simulink model "Madgwick"  (R2018a)
settings: Solver=FixedStepAuto  StartTime=0.0  StopTime=10.0  RelTol=1e-3
PreLoadFcn:
  | modelDir = fileparts(get_param(bdroot, 'FileName'));
  | addpath(fullfile(modelDir,'../../Parameters'));
  | addpath(fullfile(modelDir,'../../Estimators/Madgwick'));
  | 
  | Parameters_Estimators
  | Parameters_Simulation
InitFcn:
  | Parameters_Estimators
  | Parameters_Simulation
undefined symbols (not defined in the file or in its folder): est_q_init, Ts
settings Model: Creator=Thomas  LastModifiedBy=Thomas

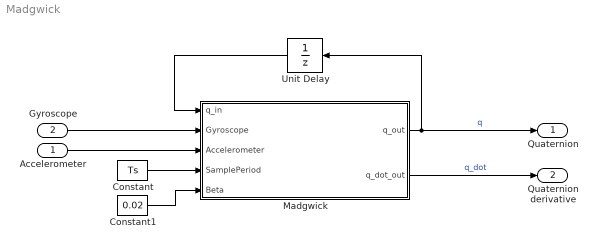
== system Madgwick ==
  Accelerometer : Inport
  Gyroscope : Inport  Port=2
  Constant : Constant  Value=Ts
  Constant1 : Constant  Value=0.02
  Madgwick : MATLAB Function  TreatAsAtomicUnit=on
  Unit Delay : UnitDelay  InitialCondition=est_q_init  SampleTime=Ts
  Quaternion : Outport
  Quaternion derivative : Outport  Port=2
  wires:
  Gyroscope/1 -> Madgwick/2(Gyroscope)
  Constant/1 -> Madgwick/4(SamplePeriod)
  Unit Delay/1 -> Madgwick/1(q_in)
  Accelerometer/1 -> Madgwick/3(Accelerometer)
  Madgwick/1(q_out) -> Unit Delay/1, Quaternion/1  "q"
  Madgwick/2(q_dot_out) -> Quaternion derivative/1  "q_dot"
  Constant1/1 -> Madgwick/5(Beta)

== matlab function Madgwick/Madgwick ==
  data: q_in input size=4; q_out output size=4; Gyroscope input size=3; Accelerometer input size=3; q_dot_out output size=4; SamplePeriod input; Beta input
function [q_out, q_dot_out] = MadgwickAHRS(q_in, Gyroscope, Accelerometer, SamplePeriod, Beta)           
    
    q = q_in';    

    % Normalise accelerometer measurement
    if(norm(Accelerometer) == 0)
        disp('ERROR - NaN in Madgwick');
        q_out = q';
        q_dot_out = [0,0,0,0]';
        return;
    end	% handle NaN
    Accelerometer = Accelerometer / norm(Accelerometer);	% normalise magnitude

    % Gradient decent algorithm corrective step
    F = [2*(q(2)*q(4) - q(1)*q(3)) - Accelerometer(1)
        2*(q(1)*q(2) + q(3)*q(4)) - Accelerometer(2)
        2*(0.5 - q(2)^2 - q(3)^2) - Accelerometer(3)];
    J = [-2*q(3),	2*q(4),    -2*q(1),	2*q(2)
        2*q(2),     2*q(1),     2*q(4),	2*q(3)
        0,         -4*q(2),    -4*q(3),	0    ];
    step = (J'*F);
    if(norm(step) == 0)
        disp('No accelerometer step taken in Madgwick');
        q_out = q';
        q_dot_out = [0,0,0,0]';                                
        return
    end
    step = step / norm(step);	% normalise step magnitude

    % Compute rate of change of quaternion
    qDot = 0.5 * quaternProd(q, [0 Gyroscope(1) Gyroscope(2) Gyroscope(3)]) - Beta * step';

    % Integrate to yield quaternion
    q = q + qDot * SamplePeriod;

    q_out = q' / norm(q); % normalise quaternion
        
    q_dot_out = qDot';
end         

function ab = quaternProd(a, b)
%QUATERNPROD Calculates the quaternion product
%
%   ab = quaternProd(a, b)
%
%   Calculates the quaternion product of quaternion a and b.
%
%   For more information see:
%   http://www.x-io.co.uk/node/8#quaternions
%
%	Date          Author          Notes
%	27/09/2011    SOH Madgwick    Initial release
    ab = zeros(1,4);
    ab(1) = a(1).*b(1)-a(2).*b(2)-a(3).*b(3)-a(4).*b(4);
    ab(2) = a(1).*b(2)+a(2).*b(1)+a(3).*b(4)-a(4).*b(3);
    ab(3) = a(1).*b(3)-a(2).*b(4)+a(3).*b(1)+a(4).*b(2);
    ab(4) = a(1).*b(4)+a(2).*b(3)-a(3).*b(2)+a(4).*b(1);
end
